simulink model "model"  (R2022a)
settings: Solver=VariableStepAuto  StartTime=0.0  StopTime=150  MaxStep=0.001  RelTol=1e-3
values from neighbouring files (symbols this model uses):
  A = double(subs(Asym))    [config.m]
  a = flip(double(coeffs(a)))    [config.m]
  B = [0;9]    [config.m]
  b = flip(double(coeffs(b)))    [config.m]
  b_0 = b(1)    [config.m]
  C = [1 0]    [config.m]
  gamma = 1000    [config.m]
  k_0 = 1    [config.m]
  Lambda = -1    [config.m]
settings Model: Creator=Vvlad  LastModifiedBy=Vvlad

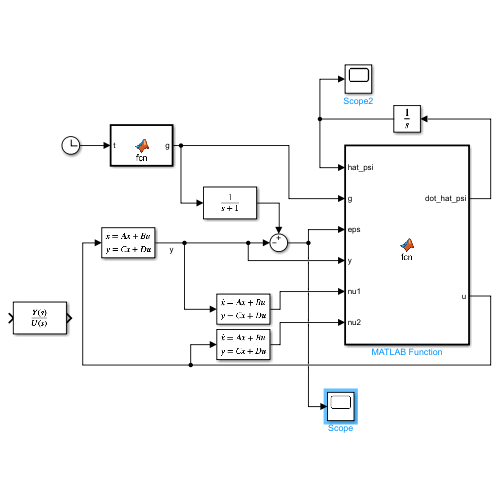
[thumbnail: Simulink's stored preview of the top-level diagram]
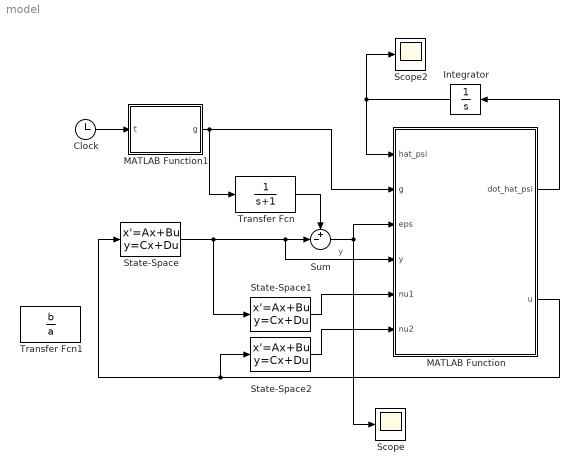
== system model ==
  Clock : Clock
  Integrator : Integrator  InitialCondition=[0; 0; 0]
  MATLAB Function : MATLAB Function  TreatAsAtomicUnit=on
  MATLAB Function1 : MATLAB Function  TreatAsAtomicUnit=on
  Scope : Scope
  Scope2 : Scope
  State-Space : StateSpace  A=A  B=B  C=C  D=0  InitialCondition=0
  State-Space1 : StateSpace  A=Lambda  D=0  InitialCondition=0
  State-Space2 : StateSpace  A=Lambda  D=0  InitialCondition=0
  Sum : Sum  Inputs=+-|
  Transfer Fcn : TransferFcn  Denominator=[1 1]
  Transfer Fcn1 : TransferFcn  Numerator=b  Denominator=a
  wires:
  State-Space1/1 -> MATLAB Function/5(nu1)
  State-Space/1 -> MATLAB Function/4(y), Sum/2, State-Space1/1  "y"
  Clock/1 -> MATLAB Function1/1(t)
  MATLAB Function1/1(g) -> Transfer Fcn/1, MATLAB Function/2(g)
  Transfer Fcn/1 -> Sum/1
  MATLAB Function/2(u) -> State-Space/1, State-Space2/1
  MATLAB Function/1(dot_hat_psi) -> Integrator/1
  Integrator/1 -> Scope2/1, MATLAB Function/1(hat_psi)
  Sum/1 -> MATLAB Function/3(eps), Scope/1
  State-Space2/1 -> MATLAB Function/6(nu2)

== matlab function model/MATLAB Function1 ==
  data: t input; g output
function g = fcn(t)

g = sin(t) + 2;

== matlab function model/MATLAB Function ==
  data: dot_hat_psi output; hat_psi input; g input; eps input; y input; u output; nu1 input; nu2 input; gamma parameter; b_0 parameter; k_0 parameter
function [dot_hat_psi, u] = fcn(hat_psi, g, eps, y, nu1, nu2, gamma, b_0, k_0)

omega = [nu1 nu2 y]';
dot_hat_psi = -gamma*omega*eps;
u = 1/b_0 * (-hat_psi'*omega + k_0*g);
